simulink model "RedCrane_kinematic_model"  (R2024a)
settings: Solver=FixedStepAuto  StartTime=0.0  StopTime=8  FixedStep=Ts  MaxStep=0.005  RelTol=1e-3
values from neighbouring files (symbols this model uses):
  M = [1, 0, 0, (L5 + L4 - L1) ... (first row only)    [enviroment_setup.m]
  SList = [ws_mat ... (first row only)    [enviroment_setup.m]
  telescope0 = 4    [enviroment_setup.m]
  thetaList0 = [0, 0, 0, 0, 0]'    [enviroment_setup.m]
  Ts = 0.001    [enviroment_setup.m]
undefined symbols (not defined in the file or in its folder): p_k_angle_to_stroke, p_k_stroke_to_angle, p_m_angle_to_stroke, p_m_stroke_to_angle, X, Y, Z
libraries: sm_lib x82, nesl_utility x19, fl_lib x16
(part 3 of 3)

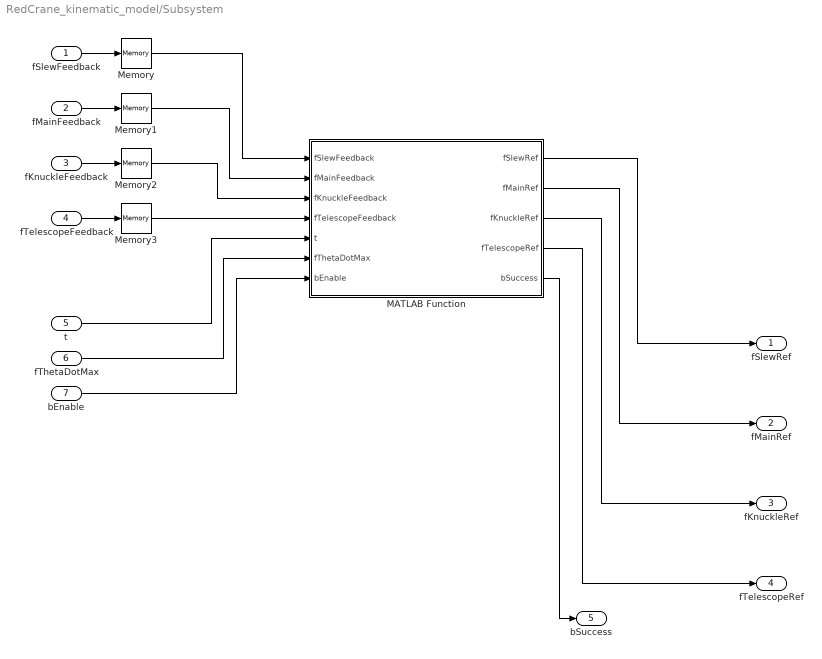
== system RedCrane_kinematic_model/Subsystem ==
  fSlewFeedback : Inport
  fMainFeedback : Inport  Port=2
  fKnuckleFeedback : Inport  Port=3
  fTelescopeFeedback : Inport  Port=4
  t : Inport  Port=5
  fThetaDotMax : Inport  Port=6
  bEnable : Inport  Port=7
  MATLAB Function : MATLAB Function  TreatAsAtomicUnit=on
  Memory : Memory  InitialCondition=thetaList0(1)
  Memory1 : Memory  InitialCondition=thetaList0(2)
  Memory2 : Memory  InitialCondition=thetaList0(3)
  Memory3 : Memory  InitialCondition=telescope0
  fSlewRef : Outport
  fMainRef : Outport  Port=2
  fKnuckleRef : Outport  Port=3
  fTelescopeRef : Outport  Port=4
  bSuccess : Outport  Port=5
  wires:
  MATLAB Function/4(fTelescopeRef) -> fTelescopeRef/1
  MATLAB Function/2(fMainRef) -> fMainRef/1
  fMainFeedback/1 -> Memory1/1
  fSlewFeedback/1 -> Memory/1
  fKnuckleFeedback/1 -> Memory2/1
  MATLAB Function/5(bSuccess) -> bSuccess/1
  t/1 -> MATLAB Function/5(t)
  MATLAB Function/1(fSlewRef) -> fSlewRef/1
  MATLAB Function/3(fKnuckleRef) -> fKnuckleRef/1
  fThetaDotMax/1 -> MATLAB Function/6(fThetaDotMax)
  bEnable/1 -> MATLAB Function/7(bEnable)
  fTelescopeFeedback/1 -> Memory3/1
  Memory/1 -> MATLAB Function/1(fSlewFeedback)
  Memory1/1 -> MATLAB Function/2(fMainFeedback)
  Memory2/1 -> MATLAB Function/3(fKnuckleFeedback)
  Memory3/1 -> MATLAB Function/4(fTelescopeFeedback)

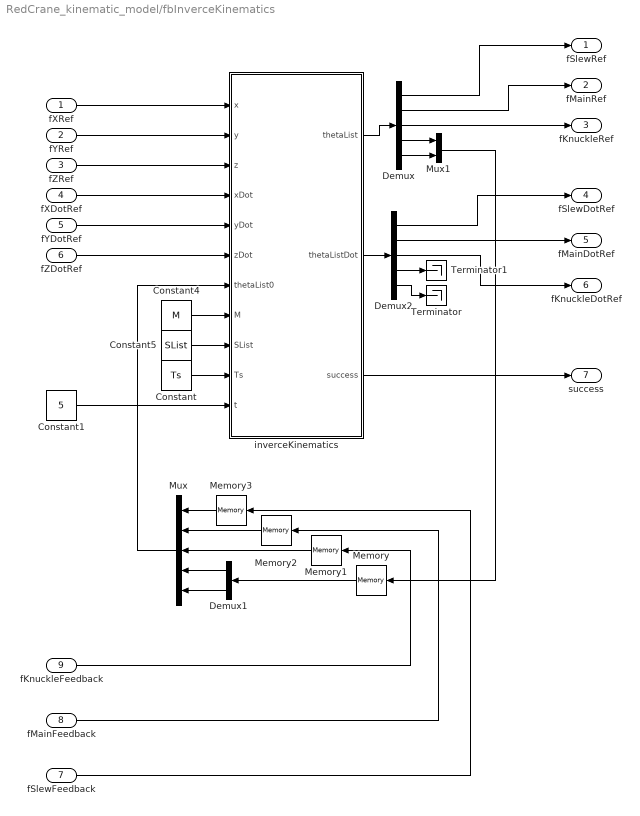
== system RedCrane_kinematic_model/fbInverceKinematics ==
  fXRef : Inport
  fYRef : Inport  Port=2
  fZRef : Inport  Port=3
  fXDotRef : Inport  Port=4
  fYDotRef : Inport  Port=5
  fZDotRef : Inport  Port=6
  fSlewFeedback : Inport  Port=7
  fMainFeedback : Inport  Port=8
  fKnuckleFeedback : Inport  Port=9
  Constant : Constant  Value=Ts
  Constant1 : Constant  Value=5
  Constant4 : Constant  Value=M
  Constant5 : Constant  Value=SList
  Demux : Demux  Outputs=5
  Demux1 : Demux  Outputs=2
  Demux2 : Demux  Outputs=5
  Memory : Memory  InitialCondition=[thetaList0(4), thetaList0(5)]'
  Memory1 : Memory  InitialCondition=thetaList0(3)
  Memory2 : Memory  InitialCondition=thetaList0(2)
  Memory3 : Memory  InitialCondition=thetaList0(1)
  Mux : Mux  Inputs=5
  Mux1 : Mux  Inputs=2
  Terminator : Terminator
  Terminator1 : Terminator
  inverceKinematics : MATLAB Function  TreatAsAtomicUnit=on
  fSlewRef : Outport
  fMainRef : Outport  Port=2
  fKnuckleRef : Outport  Port=3
  fSlewDotRef : Outport  Port=4
  fMainDotRef : Outport  Port=5
  fKnuckleDotRef : Outport  Port=6
  success : Outport  Port=7
  wires:
  Memory1/1 -> Mux/3
  Demux/5 -> Mux1/2
  Constant4/1 -> inverceKinematics/8(M)
  Memory3/1 -> Mux/1
  Demux2/5 -> Terminator/1
  fSlewFeedback/1 -> Memory3/1
  Demux1/2 -> Mux/5
  Memory2/1 -> Mux/2
  Constant5/1 -> inverceKinematics/9(SList)
  Demux2/1 -> fSlewDotRef/1
  fXDotRef/1 -> inverceKinematics/4(xDot)
  inverceKinematics/1(thetaList) -> Demux/1
  Constant1/1 -> inverceKinematics/11(t)
  Demux/1 -> fSlewRef/1
  fXRef/1 -> inverceKinematics/1(x)
  Constant/1 -> inverceKinematics/10(Ts)
  Demux1/1 -> Mux/4
  Mux/1 -> inverceKinematics/7(thetaList0)
  Mux1/1 -> Memory/1
  fZRef/1 -> inverceKinematics/3(z)
  Memory/1 -> Demux1/1
  inverceKinematics/2(thetaListDot) -> Demux2/1
  Demux/4 -> Mux1/1
  Demux2/4 -> Terminator1/1
  fMainFeedback/1 -> Memory2/1
  fYRef/1 -> inverceKinematics/2(y)
  fKnuckleFeedback/1 -> Memory1/1
  Demux/3 -> fKnuckleRef/1
  fYDotRef/1 -> inverceKinematics/5(yDot)
  fZDotRef/1 -> inverceKinematics/6(zDot)
  Demux2/3 -> fKnuckleDotRef/1
  Demux/2 -> fMainRef/1
  Demux2/2 -> fMainDotRef/1
  inverceKinematics/3(success) -> success/1

== matlab function RedCrane_kinematic_model/Subsystem/MATLAB Function ==
  settings: updateMethod=DISCRETE
  data: fSlewFeedback input; fSlewRef output; fMainRef output; fKnuckleRef output; fTelescopeRef output; fMainFeedback input; fKnuckleFeedback input; fTelescopeFeedback input; t input; bSuccess output; fThetaDotMax input; bEnable input
function [fSlewRef, fMainRef, fKnuckleRef, fTelescopeRef, bSuccess] = ...
                    goHome(fSlewFeedback, ...
                    fMainFeedback, ...
                    fKnuckleFeedback, ...
                    fTelescopeFeedback, ...
                    t,...
                    fThetaDotMax, ...
                    bEnable)
bSuccess = false;


%fSlewRef = 0;
%fMainRef = 0;
%fKnuckleRef = 0;
%fTelescopeRef = 0;

slewHomeTheta = 0.0;
mainHomeTheta = 0.0;
knuckleHomeTheta = 0.0;
telescopeHomeTheta = 2.0;


[fSlewRef, ~, bSlewDone, ~] = cosinePositionGenerator(fSlewFeedback, slewHomeTheta, fThetaDotMax, t, bEnable);
[fMainRef, ~, bMainDone, ~] = cosinePositionGenerator(fMainFeedback, mainHomeTheta, fThetaDotMax, t, bEnable);
[fKnuckleRef, ~, bKnuckleDone, ~] = cosinePositionGenerator(fKnuckleFeedback, knuckleHomeTheta, fThetaDotMax, t, bEnable);

[fTelescopeRef, ~, bTelescopeDone, ~] = cosinePositionGenerator(fTelescopeFeedback, telescopeHomeTheta, fThetaDotMax, t, bEnable);

if (bSlewDone & bMainDone & bKnuckleDone & bTelescopeDone)
    bSuccess = true;
end



end

== matlab function RedCrane_kinematic_model/fbInverceKinematics/inverceKinematics ==
  data: x input; thetaList output size=[5, 1]; y input; z input; xDot input; yDot input; zDot input; thetaList0 input; M input; SList input; Ts input; thetaListDot output size=[5, 1]; success output size=1; t input
function [thetaList, thetaListDot, success] = inverceKinematics( ...
    x, y, z, xDot, yDot, zDot, thetaList0, M, SList, Ts, t)

if(t <= Ts*1.1)
    thetaList0 = [0, 0, 0, 0, 0]';
end

% Explicitly pre-assign outputs
thetaList    = zeros(5,1);
thetaListDot = zeros(5,1);
success      = false;    % or 0 if you prefer numeric


T = [1 0 0 x;
    0 1 0 y;
    0 0 1 z;
    0 0 0 1];


[thetaOut, successOut] = IKinSpace(SList, M, T, thetaList0, 0.00001, 0.0000001);

% Assign them to the pre-allocated outputs
thetaList    = thetaOut;
success      = successOut;


Js = JacobianSpace(SList,thetaList);
Js_pinv = pinv(Js);
xyzDot = [0;
         0;
         0;
         xDot;
         yDot;
         zDot
         ];

thetaListDot = Js_pinv*xyzDot;

end

== matlab function RedCrane_kinematic_model/MATLAB Function3 ==
  data: x output; y output; z output; t_current input; x_t output; y_t output; z_t output
function [x, y, z, x_t, y_t, z_t] = CubicPlanner(t_current)

% Position (xyz) and time vectors
px = [4.55, 0, 2];
py = [0.4, 3, 1];
pz = [1.6,  1.6,  2];
t =  [0,  5,  8];

%palpha = [0 0 0 0 pi/4 0 0];

pt = [px; py; pz]';

v = 0.005;

vx = [0 v 0];
vy = [0 v 0];
vz = [0 v 0];

if(t_current < t(2))
    idx = 1;
elseif(t_current < t(3))
    idx = 2;
else
    idx = 2;
end


t0 = t(idx);

x0 = pt(idx,  1);
x1 = pt(idx+1,1);
y0 = pt(idx,  2);
y1 = pt(idx+1,2);
z0 = pt(idx,  3);
z1 = pt(idx+1,3);

v0_x = vx(idx);
v1_x = vx(idx+1);

v0_y = vy(idx);
v1_y = vy(idx+1);

v0_z = vz(idx);
v1_z = vz(idx+1);

%alpha0 = palpha(idx);
%alpha1 = palpha(idx+1);

t1 = t(idx+1);
if(t_current < t(length(px)))
[x, x_t] = CubicRT(t0, t1, t_current, x0, x1, v0_x, v1_x);
[y, y_t] = CubicRT(t0, t1, t_current, y0, y1, v0_y, v1_y);
[z, z_t] = CubicRT(t0, t1, t_current, z0, z1, v0_z, v1_z);
%[alpha, alpha_t] = QuinticRT(t0, t1, t_current, alpha0, alpha1, 0, 0.001);
else
x = px(length(px));
y = py(length(py));
z = pz(length(pz));
x_t = 0;
y_t = 0;
z_t = 0;
%alpha_t = 0;
end
